simulink model "Funcion_de_trasnferencia"  (R2024b)
settings: Solver=VariableStepAuto  StartTime=0.0  StopTime=10.0  RelTol=1e-3

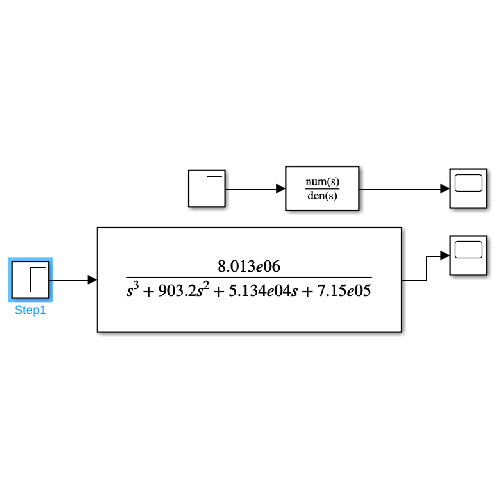
[thumbnail: Simulink's stored preview of the top-level diagram]
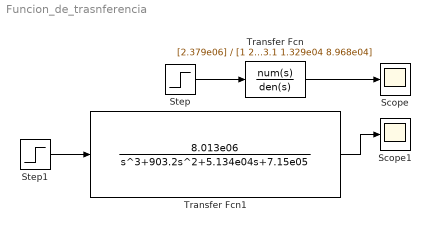
== system Funcion_de_trasnferencia ==
  Scope : Scope
  Scope1 : Scope
  Step : Step  Time=0  After=5  SampleTime=0
  Step1 : Step  Time=0  After=6  SampleTime=0
  Transfer Fcn : TransferFcn  Numerator=[2.379e06]  Denominator=[1 283.1 1.329e04 8.968e04]
  Transfer Fcn1 : TransferFcn  Numerator=[8.013e06]  Denominator=[1 903.2 5.134e04 7.15e05]
  wires:
  Step/1 -> Transfer Fcn/1
  Transfer Fcn/1 -> Scope/1
  Transfer Fcn1/1 -> Scope1/1
  Step1/1 -> Transfer Fcn1/1
